simulink model "Loss_BuckConverter"  (Simulink 7.8)
settings: Solver=ode23tb  StartTime=0.0  StopTime=4  FixedStep=1e-6  MaxStep=100e-6  RelTol=1e-4
StopFcn:
  | if OverTemp==1
  |      load explosion_sound;
  |      sound(explosion,Fs);
  | end
libraries: powerlib x11, fl_lib x8, powerlib_extras x4, nesl_utility x3, LossModelib x1, simulink x1
settings Model: Creator=Proprietaire  LastModifiedBy=at4494
settings DataIOCC: LimitDataPoints=off  SaveOutput=off  SignalLogging=off  DSMLogging=off  SaveTime=off
settings DebuggingCC: SolverPrmCheckMsg=none
settings SimscapeCC: ExplicitSolverDiagnosticOptions=none

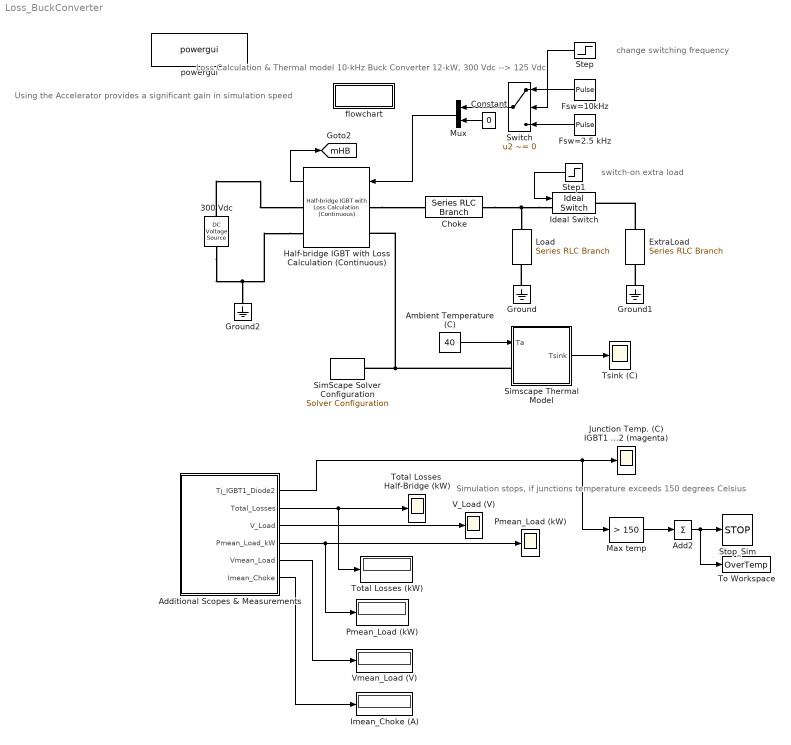
== system Loss_BuckConverter ==
  note: Loss Calculation & Thermal model
      | 10-kHz Buck Converter
      | 12-kW, 300 Vdc --> 125 Vdc
  note: switch-on extra load
  note: change switching frequency
  note: Simulation stops, if junctions temperature
      | exceeds 150 degrees Celsius
  note: Using the Accelerator provides a
      | significant gain in simulation speed
  "300 Vdc " : powerlib/Electrical Sources/DC Voltage Source  Description=source block  Amplitude=300  Measurements=None
      settings: AttributesFormatString=\n
  Add2 : Sum  Inputs=+  OutDataTypeStr=double
  Additional Scopes & Measurements : Subsystem
  Ambient Temperature (C) : Constant  Value=40
  Choke : powerlib/Elements/Series RLC Branch  LConnTagsString=__new0  RConnTagsString=__new0  BranchType=RL  Resistance=10e-3  Inductance=3e-3  SetiL0=off  InitialCurrent=100  Capacitance=1e-6  Setx0=off  InitialVoltage=0  Measurements=Branch current
  Constant : Constant  Value=0
  ExtraLoad : powerlib/Elements/Series RLC Branch  LConnTagsString=__new0  RConnTagsString=__new0  BranchType=R  Resistance=125^2/2.5e3  Inductance=1e-3  SetiL0=off  InitialCurrent=0  Capacitance=100e-6  Setx0=off  InitialVoltage=0  Measurements=Branch voltage and current
  Fsw=10kHz : DiscretePulseGenerator  PulseType=Time based  Period=1/10e3  PulseWidth=42
  Fsw=2.5 kHz : DiscretePulseGenerator  PulseType=Time based  Period=1/2.5e3  PulseWidth=42
  Ground : powerlib/Elements/Ground  LConnTagsString=a
  Ground1 : powerlib/Elements/Ground  LConnTagsString=a
  Ground2 : powerlib/Elements/Ground  LConnTagsString=a
  Half-bridge IGBT with Loss Calculation (Continuous) : LossModelib/Half-bridge IGBT with Loss Calculation (Continuous)  Ron=1e-3  IGBT_Type=Fuji: Half-bridge IGBT 600V/150A  PlotSpec_IGBT_On=off  ShowDataSheet_IGBT_On=off  Diode_Type=Fuji: Half-bridge IGBT 600V/150A  PlotSpec_Diode_On=off  ShowDataSheet_Diode_On=off  Tj_Init=40  PulseDuration=1e-6
  Ideal Switch : powerlib/Power Electronics/Ideal Switch  Ron=0.001  Lon=0  IC=0  Rs=1e5  Cs=inf  Measurements=off
  "Imean_Choke (A) " : Display
      settings: Format=bank  Decimation=3000
  Junction Temp. (C) IGBT1 and Diode2 (magenta) : Scope
      settings: TimeRange=4  YMin=40  YMax=160  SaveName=Tj_SPS_continuous  MaxDataPoints=500000  Decimation=100
  Load : powerlib/Elements/Series RLC Branch  LConnTagsString=__new0  RConnTagsString=__new0  BranchType=R  Resistance=125^2/12e3  Inductance=1e-3  SetiL0=off  InitialCurrent=0  Capacitance=100e-6  Setx0=off  InitialVoltage=0  Measurements=Branch voltage and current
  Max temp : simulink/Logic and Bit Operations/Compare To Constant  relop=>  const=150  OutDataTypeStr=uint8
  Mux : Mux  Inputs=2
  Pmean_Load (kW) : Scope
      settings: TimeRange=4  YMin=10  YMax=15  SaveName=Pmean_Load_SPS_continuous  MaxDataPoints=500000  Decimation=100
  "Pmean_Load (kW) " : Display
      settings: Format=bank  Decimation=3000
  SimScape Solver Configuration : nesl_utility/Solver Configuration  PhysicalDomain=network_engine_domain  LeftPortType=input  RightPortType=generic  SubClassName=solver  DoDC=off  ResidualTolerance=1e-9  UseLocalSolver=on  LocalSolverChoice=NE_TRAPEZOIDAL_ADVANCER  LocalSolverSampleTime=100e-6  DoFixedCost=off  MaxNonlinIter=2  MaxModeIter=1  LinearAlgebra=Sparse  Accelerate=off  Profile=off  UseLocalSampling=off  DelaysMemoryBudget=1024
  Simscape Thermal Model : Subsystem  mask(Simscape Thermal model (2-cell Cauer network)){Rth=[ 0.05  0.125 ], Cth=[ 0.25  0.25 ], Tinit=40}
      mask prompts: Rth "Thermal resistances  [case-to-sink  sink-to-ambient ] (K/W):"; Cth "Thermal capacitances  [case  sink ] (J/K):"; Tinit "Initial temperature (degrees Celsius)"
  Step : Step  Time=2.5  Before=1  After=0  SampleTime=0
  Step1 : Step  Time=2.0  SampleTime=0
  Stop_Sim : Stop
  Switch : Switch  Criteria=u2 ~= 0  Threshold=0.5
  To Workspace : ToWorkspace  VariableName=OverTemp  SampleTime=-1  SaveFormat=Array
      settings: MaxDataPoints=1
  Total Losses  Half-Bridge (kW) : Scope
      settings: TimeRange=4  YMin=0  YMax=0.35  SaveName=Total_Losses_HalfBridge  MaxDataPoints=500000  Decimation=100
  Total Losses (kW) : Display
      settings: Format=bank  Decimation=3000
  Tsink (C) : Scope
      settings: TimeRange=4  YMin=40  YMax=80  SaveName=Va_Load1  MaxDataPoints=500000  Decimation=10
  V_Load (V) : Scope
      settings: TimeRange=4  YMin=115  YMax=140  SaveName=Vload_SPS_continuous  MaxDataPoints=500000
  Vmean_Load (V) : Display
      settings: Format=bank  Decimation=3000
  flowchart : Subsystem
      settings: OpenFcn=winopen('Loss_BuckConverter_Help.pdf');
      mask Display: disp('HELP')
  powergui : powerlib/powergui  Priority=1  SimulationMode=Continuous  SolverType=Tustin  SampleTime=50e-6  frequency=60  SPID=on  DisableSnubberDevices=on  DisableRonSwitches=off  DisableVfSwitches=on  SwTol=0  Interpol=off  DisplayEquations=off  FunctionMessages=off  frequencyindice=0  Pbase=100e6  ErrMax=1e-4  Iterations=50  UnitsV=kV  UnitsW=MW  echomessages=off  HookPort=off  EnableUseOfTLC=off  x0status=blocks  RestoreLinks=warning  ResistiveCurrentMeasurement=off  Ylog=off  Xlog=on  ShowGrid=off  save=off  variable=ZData  structure=Vab_Inv  ZoomFFT=off  StartTime=4.5  cycles=3  DisplayStyle=1  fundamental=50  FreqAxis=off  MaxFrequency=5000  frequencyindicesteady=1  display=off  methode=off
  tag scope: mHB=global
  wires:
  Half-bridge IGBT with Loss Calculation (Continuous)/1 -> [mHB]
  Ambient Temperature (C)/1 -> Simscape Thermal Model/1(Ta)
  Simscape Thermal Model/1(Tsink) -> Tsink (C)/1
  Additional Scopes & Measurements/2(Total_Losses) -> Total Losses  Half-Bridge (kW)/1, Total Losses (kW)/1
  Additional Scopes & Measurements/3(V_Load) -> V_Load (V)/1
  Additional Scopes & Measurements/1(Tj_IGBT1_Diode2) -> Junction Temp. (C) IGBT1 and Diode2 (magenta)/1, Max temp/1
  Additional Scopes & Measurements/4(Pmean_Load_kW) -> "Pmean_Load (kW) "/1, Pmean_Load (kW)/1
  Additional Scopes & Measurements/5(Vmean_Load) -> Vmean_Load (V)/1
  Additional Scopes & Measurements/6(Imean_Choke) -> "Imean_Choke (A) "/1
  Step1/1 -> Ideal Switch/1
  Constant/1 -> Mux/2
  Switch/1 -> Mux/1
  Mux/1 -> Half-bridge IGBT with Loss Calculation (Continuous)/1
  Fsw=10kHz/1 -> Switch/1
  Fsw=2.5 kHz/1 -> Switch/3
  Step/1 -> Switch/2
  Max temp/1 -> Add2/1
  Add2/1 -> Stop_Sim/1, To Workspace/1
  connections:
  "300 Vdc "/RConn1 -- Half-bridge IGBT with Loss Calculation (Continuous)/RConn1
  Half-bridge IGBT with Loss Calculation (Continuous)/RConn2 -- "300 Vdc "/LConn1 -- Ground2/LConn1
  Half-bridge IGBT with Loss Calculation (Continuous)/LConn1 -- Choke/LConn1
  Ideal Switch/LConn1 -- Choke/RConn1 -- Load/LConn1
  Ground/LConn1 -- Load/RConn1
  Half-bridge IGBT with Loss Calculation (Continuous)/LConn2 -- Simscape Thermal Model/LConn1 -- SimScape Solver Configuration/RConn1
  Ground1/LConn1 -- ExtraLoad/RConn1
  ExtraLoad/LConn1 -- Ideal Switch/RConn1

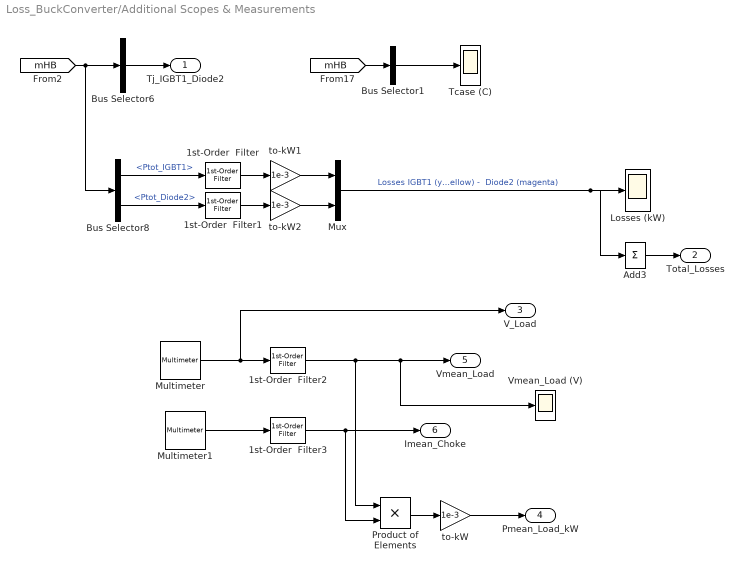
== system Loss_BuckConverter/Additional Scopes & Measurements ==
  1st-Order  Filter{,1..3} (4 alike) : powerlib_extras/Control  Blocks/1st-Order  Filter  FilterType=Lowpass  Tc=20e-3  Initialize=off  Vac_Init=[0.8 -25 60]  Vdc_Init=-0.4  PlotResponse=off  param1=[1 500 1]
  Add3 : Sum  Inputs=+
  Bus Selector1 : BusSelector  OutputSignals=Tcase  OutputAsBus=on
  Bus Selector6 : BusSelector  OutputSignals=Tj_IGBT1,Tj_Diode2  OutputAsBus=on
  Bus Selector8 : BusSelector  OutputSignals=Ptot_IGBT1,Ptot_Diode2
  Losses (kW) : Scope
      settings: TimeRange=4  YMin=0  YMax=0.2  SaveName=Losses_Continuous  MaxDataPoints=500000  Decimation=100
  Multimeter : powerlib/Measurements/Multimeter  PhasorSimulation=off  OutputType=Complex  sel=2  L=5  Gain=1  yselected={'Ub: Load'};  PSBOutputType=1  PSBequivalent=0  AxesSetting=[0,0.1,-100,100]  Display=0  SavedBlockNames=-11
  Multimeter1 : powerlib/Measurements/Multimeter  PhasorSimulation=off  OutputType=Complex  sel=3  L=5  Gain=1  yselected={'Ib: Choke'};  PSBOutputType=1  PSBequivalent=0  AxesSetting=[0,0.1,-100,100]  Display=0  SavedBlockNames=-11
  Mux : Mux  Inputs=2
  Product of Elements : Product  Inputs=**
  Tcase (C) : Scope
      settings: TimeRange=4  YMin=40  YMax=100  SaveName=psb1phPWM2_str2  MaxDataPoints=500000  Decimation=100
  Vmean_Load (V) : Scope
      settings: TimeRange=4  YMin=110.6172839506173  YMax=135.7197086282959  SaveName=Vload_Continuous1  MaxDataPoints=500000  Decimation=100
  to-kW : Gain  Gain=1e-3
  to-kW1 : Gain  Gain=1e-3
  to-kW2 : Gain  Gain=1e-3
  Tj_IGBT1_Diode2 : Outport
  Total_Losses : Outport  Port=2
  V_Load : Outport  Port=3
  Pmean_Load_kW : Outport  Port=4
  Vmean_Load : Outport  Port=5
  Imean_Choke : Outport  Port=6
  wires:
  Bus Selector1/1 -> Tcase (C)/1
  [mHB] -> Bus Selector1/1
  [mHB] -> Bus Selector6/1, Bus Selector8/1
  Bus Selector8/1 -> 1st-Order  Filter/1  "<Ptot_IGBT1>"
  Bus Selector8/2 -> 1st-Order  Filter1/1  "<Ptot_Diode2>"
  Mux/1 -> Losses (kW)/1, Add3/1  "Losses IGBT1 (yellow) -  Diode2 (magenta)"
  Add3/1 -> Total_Losses/1
  Multimeter/1 -> V_Load/1, 1st-Order  Filter2/1
  Product of Elements/1 -> to-kW/1
  Bus Selector6/1 -> Tj_IGBT1_Diode2/1
  to-kW1/1 -> Mux/1
  to-kW2/1 -> Mux/2
  to-kW/1 -> Pmean_Load_kW/1
  1st-Order  Filter/1 -> to-kW1/1
  1st-Order  Filter1/1 -> to-kW2/1
  1st-Order  Filter3/1 -> Imean_Choke/1, Product of Elements/2
  1st-Order  Filter2/1 -> Product of Elements/1, Vmean_Load/1, Vmean_Load (V)/1
  Multimeter1/1 -> 1st-Order  Filter3/1

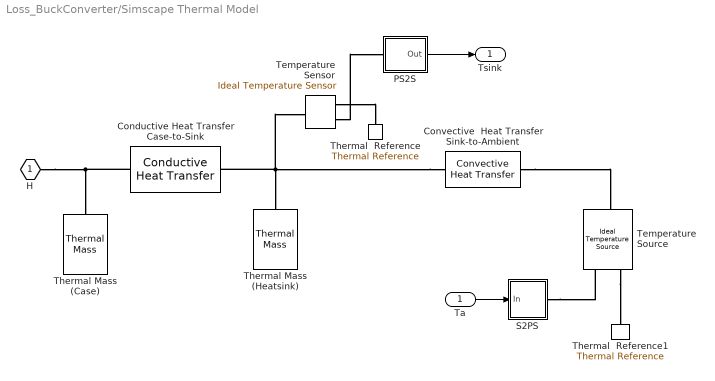
== system Loss_BuckConverter/Simscape Thermal Model ==
  Ta : Inport
  Conductive Heat Transfer Case-to-Sink : fl_lib/Thermal/Thermal Elements/Conductive Heat Transfer  area=1 m^2  thickness=1 m  th_cond=1/Rth(1) W/(m*K)  Q_Log=off  T_Log=off  LocalVarNames=|Q|T  LocalVarDescs=|Q|T  LocalVarLogging=[0 0]
  Convective  Heat Transfer Sink-to-Ambient : fl_lib/Thermal/Thermal Elements/Convective Heat Transfer  area=1 m^2  heat_tr_coeff=1/Rth(2) W/(m^2 * K)  Q_Log=off  T_Log=off  LocalVarNames=|Q|T  LocalVarDescs=|Q|T  LocalVarLogging=[0 0]
  PS2S : Subsystem
  S2PS : Subsystem
  Temperature Sensor : fl_lib/Thermal/Thermal Sensors/Ideal Temperature Sensor  Qs_Log=off  Ts_Log=off  LocalVarNames=|Qs|Ts  LocalVarDescs=|Qs|Ts  LocalVarLogging=[0 0]
  Temperature Source : fl_lib/Thermal/Thermal Sources/Ideal Temperature Source  Q_Log=off  T_Log=off  LocalVarNames=|Q|T  LocalVarDescs=|Q|T  LocalVarLogging=[0 0]
  Thermal  Reference : fl_lib/Thermal/Thermal Elements/Thermal Reference  Q_Log=off  LocalVarNames=|Q  LocalVarDescs=|Q  LocalVarLogging=0
  Thermal  Reference1 : fl_lib/Thermal/Thermal Elements/Thermal Reference  Q_Log=off  LocalVarNames=|Q  LocalVarDescs=|Q  LocalVarLogging=0
  Thermal Mass (Case) : fl_lib/Thermal/Thermal Elements/Thermal Mass  mass=Cth(1) kg  sp_heat=1 J/kg/K  init_temp=Tinit C  Q_Log=off  LocalVarNames=|Q  LocalVarDescs=|Q  LocalVarLogging=0
  Thermal Mass (Heatsink) : fl_lib/Thermal/Thermal Elements/Thermal Mass  mass=Cth(2) kg  sp_heat=1 J/kg/K  init_temp=Tinit C  Q_Log=off  LocalVarNames=|Q  LocalVarDescs=|Q  LocalVarLogging=0
  H : PMIOPort  Port=1  Side=Left
  Tsink : Outport
  wires:
  Ta/1 -> S2PS/1(In)
  PS2S/1(Out) -> Tsink/1
  connections:
  H/RConn1 -- Thermal Mass (Case)/LConn1 -- Conductive Heat Transfer Case-to-Sink/LConn1
  Temperature Source/RConn2 -- Thermal  Reference1/LConn1
  S2PS/RConn1 -- Temperature Source/RConn1
  Convective  Heat Transfer Sink-to-Ambient/RConn1 -- Temperature Source/LConn1
  Convective  Heat Transfer Sink-to-Ambient/LConn1 -- Conductive Heat Transfer Case-to-Sink/RConn1 -- Thermal Mass (Heatsink)/LConn1 -- Temperature Sensor/LConn1
  Temperature Sensor/RConn1 -- Thermal  Reference/LConn1
  Temperature Sensor/RConn2 -- PS2S/LConn1

== system Loss_BuckConverter/flowchart ==

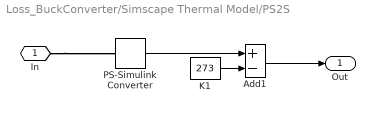
== system Loss_BuckConverter/Simscape Thermal Model/PS2S ==
  Add1 : Sum  Inputs=+-
  K1 : Constant  Value=273
  PS-Simulink Converter : nesl_utility/PS-Simulink Converter  PhysicalDomain=network_engine_domain  LeftPortType=input  RightPortType=output  SubClassName=ps_output  Unit=1  AffineConversion=off
  In : PMIOPort  Port=1  Side=Left
  Out : Outport
  wires:
  Add1/1 -> Out/1
  PS-Simulink Converter/1 -> Add1/1
  K1/1 -> Add1/2
  connections:
  In/RConn1 -- PS-Simulink Converter/LConn1

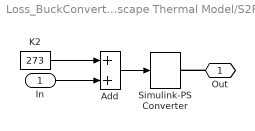
== system Loss_BuckConverter/Simscape Thermal Model/S2PS ==
  In : Inport
  Add : Sum
  K2 : Constant  Value=273
  Simulink-PS Converter : nesl_utility/Simulink-PS Converter  PhysicalDomain=network_engine_domain  LeftPortType=input  RightPortType=output  SubClassName=ps_input  Unit=1  AffineConversion=off  InputFilterTimeConstant=1e-4  UdotUserProvided=0
  Out : PMIOPort  Port=1  Side=Right
  wires:
  In/1 -> Add/2
  K2/1 -> Add/1
  Add/1 -> Simulink-PS Converter/1
  connections:
  Out/RConn1 -- Simulink-PS Converter/RConn1
